simulink model "orthographic_projection_tb"  (R2018b)
settings: Solver=FixedStepDiscrete  StartTime=0.0  StopTime=inf  FixedStep=1  RelTol=1e-3
values from neighbouring files (symbols this model uses):
  lambda0Val = cast(lambda0,'like',lambdaVec)    [test_orthographic_projection.m]    (also in test_orthographic_projection_sf.m)
  lambdaVec = fi(lambdaGr(:), dt, hdlfimath)    [test_orthographic_projection.m]    (also in test_orthographic_projection_sf.m)
  nIters = wl - 1    (= 23)    [test_orthographic_projection.m]    (also in test_orthographic_projection_sf.m)
  numSamples = n*m    (= 100)    [test_orthographic_projection.m]    (also in test_orthographic_projection_sf.m)
  phi0Val = cast(phi0,'like',phiVec)    [test_orthographic_projection.m]    (also in test_orthographic_projection_sf.m)
  phiVec = fi(phiGr(:), dt, hdlfimath)    [test_orthographic_projection.m]    (also in test_orthographic_projection_sf.m)
  RE = fi(6.371e3, 1, wl, 5)    [test_orthographic_projection.m]    (also in test_orthographic_projection_sf.m)
libraries: cordic_rotation_mode x2, simulink x1, hdlsllib x1
settings Model: DataTypeOverride=Off  Creator=jimjoy  LastModifiedBy=tbryan
settings DataIOCC: SaveFormat=StructureWithTime  SaveOutput=off  DSMLogging=off  SaveTime=off  ReturnWorkspaceOutputs=on
settings OptimizationCC: BlockReduction=off  ConditionallyExecuteInputs=off  DefaultParameterBehavior=Inlined
settings DebuggingCC: AlgebraicLoopMsg=error  SingleTaskRateTransMsg=error  UnderSpecifiedDataTypeMsg=error  UnderSpecifiedDimensionMsg=error
settings HardwareCC: ProdBitPerPointer=32  ProdBitPerSizeT=32  ProdBitPerPtrDiffT=32  ProdLargestAtomicFloat=None  ProdIntDivRoundTo=Undefined  ProdEndianess=Unspecified  ProdWordSize=32  ProdHWDeviceType=ASIC/FPGA->ASIC/FPGA  TargetBitPerLong=64  TargetBitPerPointer=64  TargetBitPerSizeT=64  TargetBitPerPtrDiffT=64  TargetLongLongMode=on  TargetIntDivRoundTo=Zero  TargetEndianess=LittleEndian  TargetWordSize=64  TargetHWDeviceType=Custom Processor->MATLAB Host Computer  ProdEqTarget=off

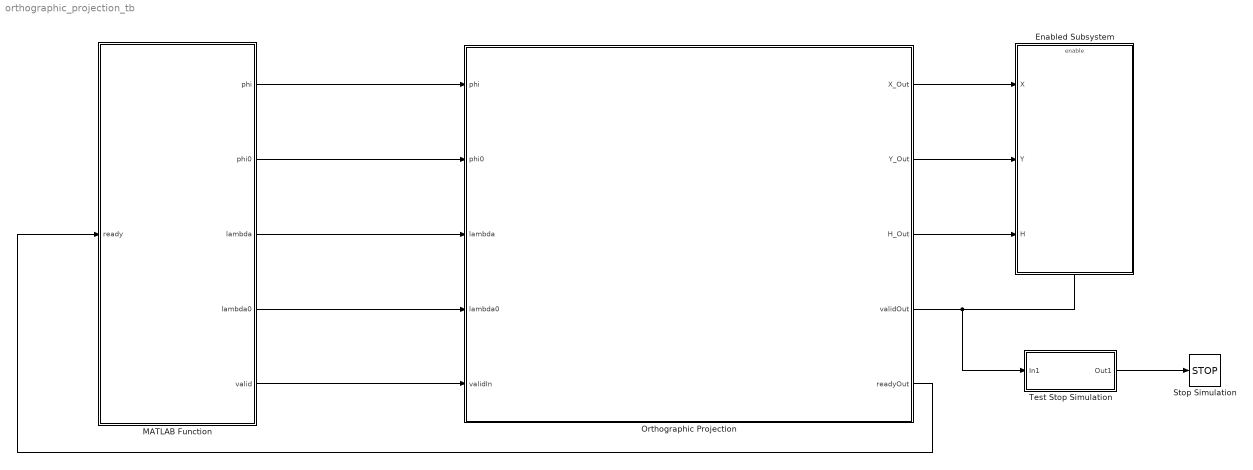
== system orthographic_projection_tb ==
  Enabled Subsystem : Subsystem  TreatAsAtomicUnit=on
  MATLAB Function : MATLAB Function  TreatAsAtomicUnit=on  mask{phiVec=phiVec, lambdaVec=lambdaVec, numSamples=numSamples, phi0Val=phi0Val, lambda0Val=lambda0Val}
      mask prompts: phiVec "phi"; lambdaVec "lambda"; numSamples "Number of Samples"; phi0Val "phi0"; lambda0Val "lambda0"
  Orthographic Projection : Subsystem
  Stop Simulation : Stop
  Test Stop Simulation : Subsystem
  wires:
  Orthographic Projection/1(X_Out) -> Enabled Subsystem/1(X)
  Orthographic Projection/2(Y_Out) -> Enabled Subsystem/2(Y)
  Orthographic Projection/3(H_Out) -> Enabled Subsystem/3(H)
  Orthographic Projection/4(validOut) -> Test Stop Simulation/1(In1), Enabled Subsystem/Enable
  Orthographic Projection/5(readyOut) -> MATLAB Function/1(ready)
  MATLAB Function/5(valid) -> Orthographic Projection/5(validIn)
  MATLAB Function/4(lambda0) -> Orthographic Projection/4(lambda0)
  MATLAB Function/3(lambda) -> Orthographic Projection/3(lambda)
  MATLAB Function/2(phi0) -> Orthographic Projection/2(phi0)
  MATLAB Function/1(phi) -> Orthographic Projection/1(phi)
  Test Stop Simulation/1(Out1) -> Stop Simulation/1

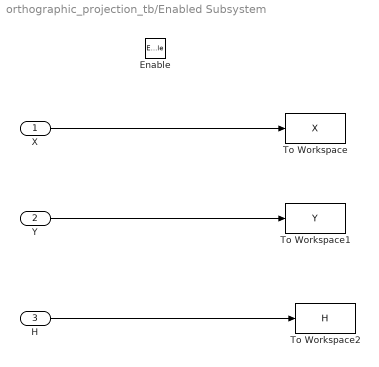
== system orthographic_projection_tb/Enabled Subsystem ==
  X : Inport
  Y : Inport  Port=2
  H : Inport  Port=3
  Enable : EnablePort
  To Workspace : ToWorkspace  VariableName=X  SampleTime=-1
      settings: Save2DSignal=2-D array (concatenate along first dimension)
  To Workspace1 : ToWorkspace  VariableName=Y  SampleTime=-1
      settings: Save2DSignal=2-D array (concatenate along first dimension)
  To Workspace2 : ToWorkspace  VariableName=H  SampleTime=-1
      settings: Save2DSignal=2-D array (concatenate along first dimension)
  wires:
  X/1 -> To Workspace/1
  Y/1 -> To Workspace1/1
  H/1 -> To Workspace2/1

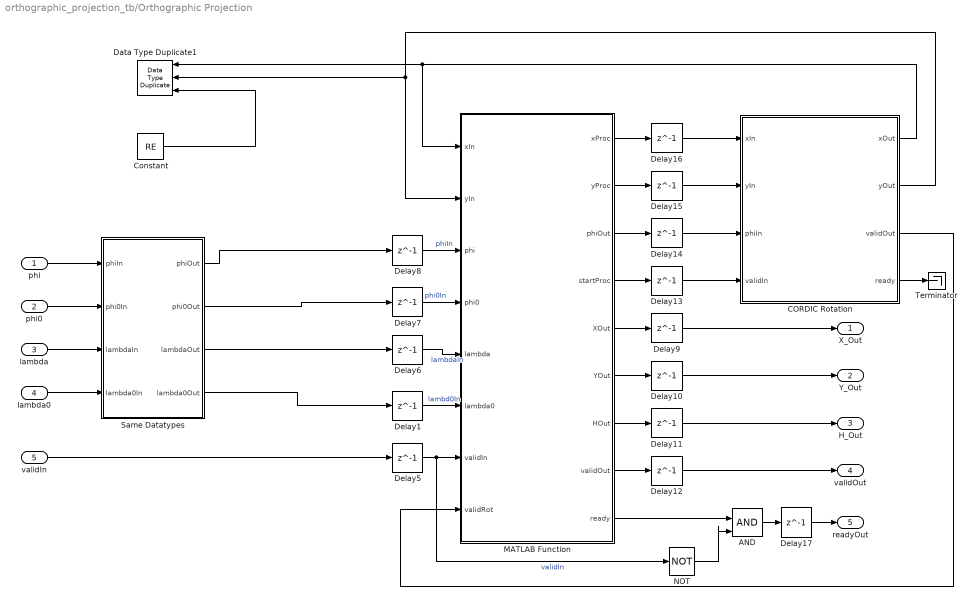
== system orthographic_projection_tb/Orthographic Projection ==
  phi : Inport
  phi0 : Inport  Port=2
  lambda : Inport  Port=3
  lambda0 : Inport  Port=4
  validIn : Inport  Port=5
  AND : Logic  IconShape=distinctive  AllPortsSameDT=off  OutDataTypeStr=boolean
  CORDIC Rotation : Subsystem
  Constant : Constant  Value=RE
  Data Type Duplicate1 : DataTypeDuplicate  NumInputPorts=3
  Delay{1,5..17} (14 alike) : Delay  DelayLength=1
  MATLAB Function : MATLAB Function  TreatAsAtomicUnit=on  mask{RE=RE}
      mask prompts: RE "Radius of the Earth"
  NOT : Logic  Operator=NOT  IconShape=distinctive  AllPortsSameDT=off  OutDataTypeStr=boolean
  Same Datatypes : Subsystem
  Terminator : Terminator
  X_Out : Outport
  Y_Out : Outport  Port=2
  H_Out : Outport  Port=3
  validOut : Outport  Port=4
  readyOut : Outport  Port=5
  wires:
  MATLAB Function/1(xProc) -> Delay16/1
  MATLAB Function/2(yProc) -> Delay15/1
  MATLAB Function/3(phiOut) -> Delay14/1
  MATLAB Function/4(startProc) -> Delay13/1
  CORDIC Rotation/1(xOut) -> MATLAB Function/1(xIn), Data Type Duplicate1/1
  CORDIC Rotation/2(yOut) -> MATLAB Function/2(yIn), Data Type Duplicate1/2
  CORDIC Rotation/3(validOut) -> MATLAB Function/8(validRot)
  MATLAB Function/5(XOut) -> Delay9/1
  MATLAB Function/6(YOut) -> Delay10/1
  MATLAB Function/7(HOut) -> Delay11/1
  MATLAB Function/8(validOut) -> Delay12/1
  lambda0/1 -> Same Datatypes/4(lambda0In)
  phi0/1 -> Same Datatypes/2(phi0In)
  lambda/1 -> Same Datatypes/3(lambdaIn)
  phi/1 -> Same Datatypes/1(phiIn)
  Same Datatypes/4(lambda0Out) -> Delay1/1
  Same Datatypes/1(phiOut) -> Delay8/1
  Same Datatypes/2(phi0Out) -> Delay7/1
  Same Datatypes/3(lambdaOut) -> Delay6/1
  validIn/1 -> Delay5/1
  Delay5/1 -> MATLAB Function/7(validIn), NOT/1  "validIn"
  Delay6/1 -> MATLAB Function/5(lambda)  "lambdaIn"
  Delay7/1 -> MATLAB Function/4(phi0)  "phi0In"
  Delay8/1 -> MATLAB Function/3(phi)  "phiIn"
  Delay13/1 -> CORDIC Rotation/4(validIn)
  Delay14/1 -> CORDIC Rotation/3(phiIn)
  Delay15/1 -> CORDIC Rotation/2(yIn)
  Delay16/1 -> CORDIC Rotation/1(xIn)
  CORDIC Rotation/4(ready) -> Terminator/1
  Delay9/1 -> X_Out/1
  Delay10/1 -> Y_Out/1
  Delay11/1 -> H_Out/1
  Delay12/1 -> validOut/1
  MATLAB Function/9(ready) -> AND/1
  NOT/1 -> AND/2
  AND/1 -> Delay17/1
  Delay17/1 -> readyOut/1
  Delay1/1 -> MATLAB Function/6(lambda0)  "lambd0In"
  Constant/1 -> Data Type Duplicate1/3

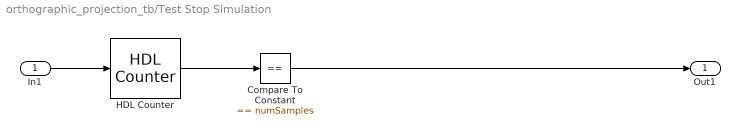
== system orthographic_projection_tb/Test Stop Simulation ==
  In1 : Inport
  Compare To Constant : simulink/Logic and Bit Operations/Compare To Constant  relop===  const=numSamples  OutDataTypeStr=boolean
  HDL Counter : hdlsllib/Sources/HDL Counter  CountType=Free running  CountInit=0  CountStep=1  CountMax=25  CountFromType=Initial value  CountFrom=0  CountResetPort=off  CountLoadPort=off  CountEnbPort=on  CountDirPort=off  CountDataType=Unsigned  CountWordLen=nextpow2(numSamples)  CountFracLen=0  CountSampTime=1
      settings: SourceProductName=Simulink
  Out1 : Outport
  wires:
  In1/1 -> HDL Counter/1
  HDL Counter/1 -> Compare To Constant/1
  Compare To Constant/1 -> Out1/1

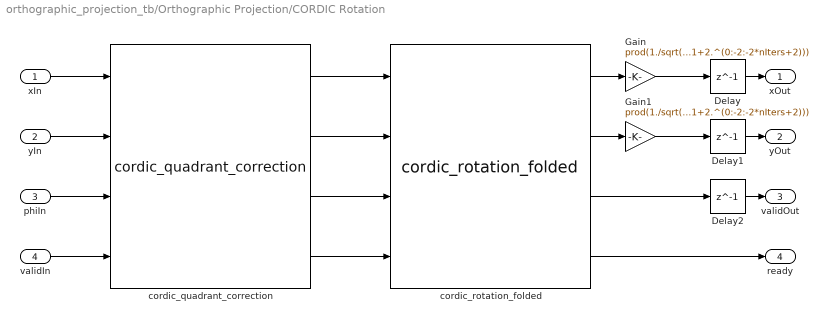
== system orthographic_projection_tb/Orthographic Projection/CORDIC Rotation ==
  xIn : Inport
  yIn : Inport  Port=2
  phiIn : Inport  Port=3
  validIn : Inport  Port=4
  Delay : Delay  DelayLength=1
  Delay1 : Delay  DelayLength=1
  Delay2 : Delay  DelayLength=1
  Gain : Gain  Gain=prod(1./sqrt(1+2.^(0:-2:-2*nIters+2)))  OutDataTypeStr=Inherit: Same as input
  Gain1 : Gain  Gain=prod(1./sqrt(1+2.^(0:-2:-2*nIters+2)))  OutDataTypeStr=Inherit: Same as input
  cordic_quadrant_correction : cordic_rotation_mode/cordic_quadrant_correction  SystemSampleTime=-1
  cordic_rotation_folded : cordic_rotation_mode/cordic_rotation_folded  nIters=nIters
  xOut : Outport
  yOut : Outport  Port=2
  validOut : Outport  Port=3
  ready : Outport  Port=4
  wires:
  Gain1/1 -> Delay1/1
  cordic_quadrant_correction/1 -> cordic_rotation_folded/1
  cordic_rotation_folded/3 -> Delay2/1
  cordic_rotation_folded/2 -> Gain1/1
  cordic_rotation_folded/1 -> Gain/1
  cordic_quadrant_correction/2 -> cordic_rotation_folded/2
  cordic_quadrant_correction/3 -> cordic_rotation_folded/3
  Gain/1 -> Delay/1
  cordic_quadrant_correction/4 -> cordic_rotation_folded/4
  xIn/1 -> cordic_quadrant_correction/1
  Delay/1 -> xOut/1
  Delay2/1 -> validOut/1
  validIn/1 -> cordic_quadrant_correction/4
  Delay1/1 -> yOut/1
  phiIn/1 -> cordic_quadrant_correction/3
  yIn/1 -> cordic_quadrant_correction/2
  cordic_rotation_folded/4 -> ready/1

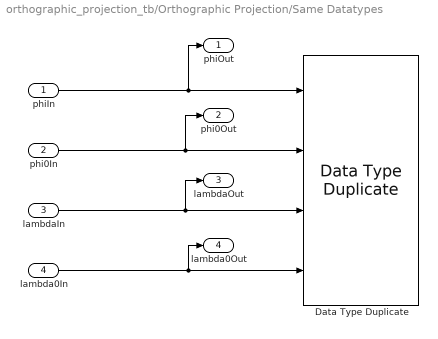
== system orthographic_projection_tb/Orthographic Projection/Same Datatypes ==
  phiIn : Inport
  phi0In : Inport  Port=2
  lambdaIn : Inport  Port=3
  lambda0In : Inport  Port=4
  Data Type Duplicate : DataTypeDuplicate  NumInputPorts=4
  phiOut : Outport
  phi0Out : Outport  Port=2
  lambdaOut : Outport  Port=3
  lambda0Out : Outport  Port=4
  wires:
  lambdaIn/1 -> lambdaOut/1, Data Type Duplicate/3
  phiIn/1 -> Data Type Duplicate/1, phiOut/1
  lambda0In/1 -> lambda0Out/1, Data Type Duplicate/4
  phi0In/1 -> phi0Out/1, Data Type Duplicate/2

== matlab function orthographic_projection_tb/MATLAB Function ==
  data: ready input; phi output; phi0 output; lambda output; lambda0 output; valid output; phiVec parameter; lambdaVec parameter; numSamples parameter; phi0Val parameter; lambda0Val parameter
function [phi, phi0, lambda, lambda0, valid] = getData(ready, phiVec, lambdaVec, numSamples, phi0Val, lambda0Val)
%#codegen

persistent ii 

if isempty(ii)
    ii = 1;
end

phi0 = phi0Val;
lambda0 = lambda0Val;
phi = phiVec(ii);
lambda = lambdaVec(ii);

if ready
   valid = true;
   if ii < numSamples
      ii = ii + 1;
   else
       ii = 1;
   end
else
    valid = false;
end

end

== matlab function orthographic_projection_tb/Orthographic Projection/MATLAB Function ==
  settings: fimath=hdlfimath
  data: xIn input; yIn input; phi input; phi0 input; xProc output size=1; lambda input; lambda0 input; validIn input; validRot input; yProc output size=1; phiOut output size=1; startProc output size=1; XOut output size=1; YOut output size=1; HOut output size=1; validOut output size=1; ready output size=1; RE parameter
function [xProc, yProc, phiOut, startProc, XOut, YOut, HOut, validOut, ready] = ...
        memctrl(xIn, yIn, phi, phi0, lambda, lambda0, validIn, validRot, RE)
    
    % Copyright 2018 The MathWorks, Inc.
    
    %#codegen
    
    % State machine used to control The CORDIC Computations for the
    % orthographic projection
    
    persistent state xReg yReg hReg
    persistent phi0Reg lambdaReg 
    persistent readyReg rotNum
    persistent bufferFull phiBuff phi0Buff lambdaBuff
    
    st = ortho.getStateTable;
    
    % Define some useful constants
    piBy2 = cast(pi/2,'like',phi);
    
    if isempty(state)
        state = st.Idle;
        xReg = cast(0,'like',RE);
        yReg = cast(0,'like',RE);
        hReg = cast(RE,'like',RE);
        phi0Reg = cast(0,'like',phi);
        lambdaReg = cast(0,'like',phi);
        readyReg = true;
        rotNum = fi(0,0,2,0);
        bufferFull = false;
        phiBuff = cast(0,'like',phi);
        phi0Buff = cast(0,'like',phi);
        lambdaBuff = cast(0,'like',phi);
    end
    
    xProc = cast(0,'like',RE);
    yProc = cast(RE,'like',RE);
    phiOut = cast(0,'like',phi);
    startProc = false;
    XOut = cast(0,'like',RE);
    YOut = cast(0,'like',RE);
    HOut = cast(0,'like',RE);
    validOut = false;
    ready = readyReg;
    
    stateNext = st.Idle;
    xRegNext = xReg;
    yRegNext = yReg;
    hRegNext = hReg;
    rotNumNext = rotNum;
    readyRegNext = false;
    phi0RegNext = cast(phi0 - piBy2,'like',phi0);
    phiNext = cast(piBy2 - phi,'like',phi);
    lambdaRegNext = cast(lambda - lambda0,'like',lambda);
    
    % Buffer logic
    nextBufferFull = bufferFull;
    nextPhiBuff = phiBuff;
    nextPhi0Buff = phi0Buff;
    nextLambdaBuff = lambdaBuff;
    if ~(bufferFull || readyReg)
        nextBufferFull(:) = validIn;
        nextPhiBuff(:) = piBy2 - phi;
        nextPhi0Buff(:) = phi0 - piBy2;
        nextLambdaBuff(:) = lambdaRegNext;
    end
    
    switch state
        case(st.Idle)
            startProc(:) = true;
            if (validIn && readyReg)
                stateNext(:) = st.Processing;
                phiOut(:) = phiNext;
            elseif bufferFull
                stateNext(:) = st.Processing;
                phiOut(:) = phiBuff;
                phi0RegNext(:) = phi0Buff;
                lambdaRegNext(:) = lambdaBuff;
                nextBufferFull(:) = false;
            else
                stateNext(:) = st.Idle;
                readyRegNext(:) = true;
                startProc(:) = false;
            end            
        case(st.Processing)
            startProc(:) = true;
            validOut(:) = false;
            phi0RegNext = phi0Reg;
            lambdaRegNext = lambdaReg;
            if validRot 
                stateNext(:) = st.Processing;
                switch rotNum
                    case(0)
                        rotNumNext(:) = rotNum + 1;
                        xProc(:) = xReg;
                        yProc(:) = xIn;
                        phiOut(:) = lambdaReg;
                        xRegNext(:) = xReg;
                        yRegNext(:) = xIn;
                        hRegNext(:) = yIn;
                    case(1)
                        rotNumNext(:) = rotNum + 1;
                        xProc(:) = yIn;
                        yProc(:) = hReg;
                        phiOut(:) = phi0Reg;
                        xRegNext(:) = xIn;
                        yRegNext(:) = yIn;
                        hRegNext(:) = hReg;
                    case(2)
                        rotNumNext(:) = 0;
                        stateNext(:) = st.Done;
                        xProc(:) = 0;
                        yProc(:) = 0;
                        startProc(:) = false;
                        validOut(:) = true;
                        XOut(:) = xReg;
                        YOut(:) = xIn;
                        HOut(:) = yIn;
                    otherwise
                        rotNumNext(:) = 0;
                        stateNext(:) = st.Idle;
                        xProc(:) = 0;
                        yProc(:) = 0;
                        startProc(:) = false;
                        validOut(:) = false;
                end
            else
                stateNext = st.Processing;
                rotNumNext(:) = rotNum;
                startProc(:) = false;
            end
        case(st.Done)
            stateNext(:) = st.Idle;
            xRegNext(:) = 0;
            yRegNext(:) = 0;
            hRegNext(:) = RE;
            readyRegNext(:) = ~bufferFull;
            rotNumNext(:) = 0;
        otherwise
            stateNext(:) = st.Idle;
            xRegNext(:) = 0;
            yRegNext(:) = 0;
            hRegNext(:) = RE;
            readyRegNext(:) = true;
            rotNumNext(:) = 0;
    end
    
    
    state(:) = stateNext;
    readyReg(:) = readyRegNext;
    phi0Reg(:) = phi0RegNext;
    lambdaReg(:) = lambdaRegNext;
    rotNum(:) = rotNumNext;
    xReg(:) = xRegNext;
    yReg(:) = yRegNext;
    hReg(:) = hRegNext;
    bufferFull(:) = nextBufferFull;
    phiBuff(:) = nextPhiBuff;
    phi0Buff(:) = nextPhi0Buff;
    lambdaBuff(:) = nextLambdaBuff;
    
    
end
